simulink subsystem "FlightControl"  (R2024b)
settings: Solver=VariableStepAuto  StartTime=0.0  StopTime=10.0  RelTol=1e-3
undefined symbols (not defined in the file): control, controlParams, ControlSampleTime, CriticalTiltAngle, DiscIntNeverNeededParam, flightState, FWControlParams, FWTrimSpeed, tilt_max, tilt_trim, TiltScheduleRate, uavParam, w_trim, WindDownRate
libraries: slpidlib x31, simulink x9
(part 5 of 5)

== matlab function FlightControl/Fixed Wing Controller/Fixed Wing Controller Module/Fixed Wing Controller Simulation/Attitude Controller/Pitch Roll Controller/Turn Coordinator/MATLAB Function ==
  data: rollSP input; rSP output; pitchSP input; airSpeed input
function rSP = fcn(rollSP, pitchSP, airSpeed)
    yawRateSP = tan(rollSP)*9.81/max(airSpeed,5);
    rSP = yawRateSP*cos(pitchSP)*cos(rollSP);
end

== matlab function FlightControl/Fixed Wing Controller/Fixed Wing Controller Module/Fixed Wing Controller Simulation/Lateral Guidance Logic/MATLAB Function ==
  data: courseSP input; lacc output; course input; rollSP output; groundSpeed input; L1 input
function [lacc, rollSP] = fcn(courseSP, course, groundSpeed, L1)
eta = courseSP - course;

% wrap -pi to pi
eta = mod(eta, 2*pi);
if eta>pi
    eta = eta - 2*pi;
end

% cap eta to -pi/2 to pi/2
eta = min(eta, pi/2);
eta = max(eta, -pi/2);

lacc = 2*(groundSpeed^2)/L1*sin(eta);

rollSP = atan(lacc/9.81);

== matlab function FlightControl/Fixed Wing Controller/Fixed Wing Controller Module/Fixed Wing Controller Simulation/Subsystem2/MATLAB Function ==
  data: phi input; y output; theta input
function y = fcn(phi,theta)

y=zeros(3,3);
y=[1 sin(phi)*tan(theta) cos(phi)*tan(theta); 0 cos(phi) -sin(phi); 0 sin(phi)/cos(theta) cos(phi)/cos(theta)];
end

== matlab function FlightControl/Fixed Wing Controller/Fixed Wing Controller Module/Fixed Wing Controller Tuning/Attitude Controller/Pitch Roll Controller/Turn Coordinator/MATLAB Function ==
  data: rollSP input; rSP output; pitchSP input; airSpeed input
function rSP = fcn(rollSP, pitchSP, airSpeed)
    yawRateSP = tan(rollSP)*9.81/max(airSpeed,5);
    rSP = yawRateSP*cos(pitchSP)*cos(rollSP);
end

== matlab function FlightControl/Fixed Wing Controller/Fixed Wing Controller Module/Fixed Wing Controller Tuning/Lateral Guidance Logic/MATLAB Function ==
  data: courseSP input; lacc output; course input; rollSP output; groundSpeed input; L1 input
function [lacc, rollSP] = fcn(courseSP, course, groundSpeed, L1)
eta = courseSP - course;

% wrap -pi to pi
eta = mod(eta, 2*pi);
if eta>pi
    eta = eta - 2*pi;
end

% cap eta to -pi/2 to pi/2
eta = min(eta, pi/2);
eta = max(eta, -pi/2);

lacc = 2*(groundSpeed^2)/L1*sin(eta);

rollSP = atan(lacc/9.81);

== matlab function FlightControl/Fixed Wing Controller/Fixed Wing Controller Module/Fixed Wing Controller Tuning/Subsystem2/MATLAB Function ==
  data: phi input; y output; theta input
function y = fcn(phi,theta)

y=zeros(3,3);
y=[1 sin(phi)*tan(theta) cos(phi)*tan(theta); 0 cos(phi) -sin(phi); 0 sin(phi)/cos(theta) cos(phi)/cos(theta)];
end
